simulink model "a1_walking_backward"  (R2022b)
settings: Solver=VariableStepAuto  StartTime=0.0  StopTime=5  RelTol=1e-3
values from neighbouring files (symbols this model uses):
  m = 12    [MPC_Controller.m]    (also in QP_Controller.m; TASK1_rotating_mpc.m; TASK1_walking_backward_mpc.m; TASK1_walking_forward_mpc.m)
  N = 10    [MPC_Controller.m]
undefined symbols (not defined in the file or in its folder): walking_forward_mpc, X, Y, Z
libraries: sm_lib x188, nesl_utility x120
(part 5 of 6)

== system a1_walking_backward/Rear Left Leg/RL_thigh ==
  Inertia : sm_lib/Body Elements/Inertia  InertiaType=Custom  Mass=1.013  MassUnits=kg  CenterOfMass=[0, 0, 0]  CenterOfMassUnits=m  MomentsOfInertia=[0.005529065, 0.005139339, 0.001367788]  MomentsOfInertiaUnits=kg*m^2  ProductsOfInertia=[2.2448e-05, 0.000343869, 4.825e-06]  ProductsOfInertiaUnits=kg*m^2  GraphicType=None  MarkerShape=Inertia  MarkerSize=20  GraphicVisPropType=SimpleVisualProperties  GraphicDiffuseColor=[0.5 0.5 0.5]  GraphicSpecularColor=[0.5 0.5 0.5 1.0]  GraphicAmbientColor=[0.15 0.15 0.15 1.0]  GraphicEmissiveColor=[0.0 0.0 0.0 1.0]  GraphicShininess=75  GraphicOpacity=1.0
  InertiaOriginTransform : sm_lib/Frames and Transforms/Rigid Transform  TranslationMethod=Cartesian  TranslationStandardOffset=0  TranslationLengthUnit=m  TranslationStandardAxis=+Z  TranslationCartesianOffset=[-0.003237, -0.022327, -0.027326]  TranslationROffset=0  TranslationROffsetUnits=m  TranslationZOffset=0  TranslationZOffsetUnits=m  TranslationThetaOffset=0  TranslationThetaOffsetUnits=deg  RotationMethod=RotationSequence  RotationAngleUnits=deg  RotationStandardAxis=+Z  RotationAngle=0.0  RotationArbitraryAxis=[0 0 1]  FollAlignAxisA=+X  BaseAlignAxisA=+Y  FollAlignAxisB=+Y  BaseAlignAxisB=+Z  RotationSequenceAxes=BaseAxes  RotationSequence=XYZ  RotationSequenceAngles=[0, 0, 0]  RotationSequenceAnglesUnits=rad  RotationMatrix=[1 0 0; 0 1 0; 0 0 1]  Quaternion=[1 0 0 0]
  RL_calf_joint_AxisTransform : sm_lib/Frames and Transforms/Rigid Transform  TranslationMethod=Cartesian  TranslationStandardOffset=0  TranslationLengthUnit=m  TranslationStandardAxis=+Z  TranslationCartesianOffset=[0, 0, 0]  TranslationROffset=0  TranslationROffsetUnits=m  TranslationZOffset=0  TranslationZOffsetUnits=m  TranslationThetaOffset=0  TranslationThetaOffsetUnits=deg  RotationMethod=ArbitraryAxis  RotationAngleUnits=rad  RotationStandardAxis=+Z  RotationAngle=1.570796326794897  RotationArbitraryAxis=[-1, 0, 0]  FollAlignAxisA=+X  BaseAlignAxisA=+Y  FollAlignAxisB=+Y  BaseAlignAxisB=+Z  RotationSequenceAxes=FollowerAxes  RotationSequence=XYX  RotationSequenceAngles=[0 0 0]  RotationSequenceAnglesUnits=deg  RotationMatrix=[1 0 0; 0 1 0; 0 0 1]  Quaternion=[1 0 0 0]
  RL_calf_joint_OriginTransform : sm_lib/Frames and Transforms/Rigid Transform  TranslationMethod=Cartesian  TranslationStandardOffset=0  TranslationLengthUnit=m  TranslationStandardAxis=+Z  TranslationCartesianOffset=[0, 0, -0.2]  TranslationROffset=0  TranslationROffsetUnits=m  TranslationZOffset=0  TranslationZOffsetUnits=m  TranslationThetaOffset=0  TranslationThetaOffsetUnits=deg  RotationMethod=RotationSequence  RotationAngleUnits=deg  RotationStandardAxis=+Z  RotationAngle=0.0  RotationArbitraryAxis=[0 0 1]  FollAlignAxisA=+X  BaseAlignAxisA=+Y  FollAlignAxisB=+Y  BaseAlignAxisB=+Z  RotationSequenceAxes=BaseAxes  RotationSequence=XYZ  RotationSequenceAngles=[0, 0, 0]  RotationSequenceAnglesUnits=rad  RotationMatrix=[1 0 0; 0 1 0; 0 0 1]  Quaternion=[1 0 0 0]
  RL_thigh_joint_AxisInvTransform : sm_lib/Frames and Transforms/Rigid Transform  TranslationMethod=Cartesian  TranslationStandardOffset=0  TranslationLengthUnit=m  TranslationStandardAxis=+Z  TranslationCartesianOffset=[0, 0, 0]  TranslationROffset=0  TranslationROffsetUnits=m  TranslationZOffset=0  TranslationZOffsetUnits=m  TranslationThetaOffset=0  TranslationThetaOffsetUnits=deg  RotationMethod=ArbitraryAxis  RotationAngleUnits=rad  RotationStandardAxis=+Z  RotationAngle=1.570796326794897  RotationArbitraryAxis=[-1, 0, 0]  FollAlignAxisA=+X  BaseAlignAxisA=+Y  FollAlignAxisB=+Y  BaseAlignAxisB=+Z  RotationSequenceAxes=FollowerAxes  RotationSequence=XYX  RotationSequenceAngles=[0 0 0]  RotationSequenceAnglesUnits=deg  RotationMatrix=[1 0 0; 0 1 0; 0 0 1]  Quaternion=[1 0 0 0]
  ReferenceFrame : sm_lib/Frames and Transforms/Reference Frame
  Visual : sm_lib/Body Elements/File Solid  ExtGeomFileName=AME556_project/a1_description/meshes/thigh.stl  UnitType=Custom  ExtGeomFileUnits=m  StepReaderType=HEX  ExportConvexHullGeometry=on  InertiaType=Custom  Mass=0  MassUnits=kg  CenterOfMass=[0, 0, 0]  CenterOfMassUnits=m  MomentsOfInertia=[0, 0, 0]  MomentsOfInertiaUnits=kg*m^2  ProductsOfInertia=[0, 0, 0]  ProductsOfInertiaUnits=kg*m^2  BasedOnType=DensityFromFile  Density=1000  DensityUnits=kg/m^3  DoExposeReferenceFrame=on  SerializedFrames=<Frames/>  GraphicType=FromGeometry  MarkerShape=Sphere  MarkerSize=10  GraphicVisPropType=SimpleVisualProperties  GraphicDiffuseColor=[1, 0.423529411765, 0.0392156862745]  GraphicSpecularColor=[0.5 0.5 0.5 1.0]  GraphicAmbientColor=[0.15 0.15 0.15 1.0]  GraphicEmissiveColor=[0.0 0.0 0.0 1.0]  GraphicShininess=75  GraphicOpacity=1
  VisualOriginTransform : sm_lib/Frames and Transforms/Rigid Transform  TranslationMethod=Cartesian  TranslationStandardOffset=0  TranslationLengthUnit=m  TranslationStandardAxis=+Z  TranslationCartesianOffset=[0, 0, 0]  TranslationROffset=0  TranslationROffsetUnits=m  TranslationZOffset=0  TranslationZOffsetUnits=m  TranslationThetaOffset=0  TranslationThetaOffsetUnits=deg  RotationMethod=RotationSequence  RotationAngleUnits=deg  RotationStandardAxis=+Z  RotationAngle=0.0  RotationArbitraryAxis=[0 0 1]  FollAlignAxisA=+X  BaseAlignAxisA=+Y  FollAlignAxisB=+Y  BaseAlignAxisB=+Z  RotationSequenceAxes=BaseAxes  RotationSequence=XYZ  RotationSequenceAngles=[0, 0, 0]  RotationSequenceAnglesUnits=rad  RotationMatrix=[1 0 0; 0 1 0; 0 0 1]  Quaternion=[1 0 0 0]
  F : PMIOPort  Side=Left
  F1 : PMIOPort  Port=2  Side=Right
  G : PMIOPort  Port=3  Side=Right
  connections:
  Inertia/RConn1 -- InertiaOriginTransform/RConn1
  RL_calf_joint_AxisTransform/RConn1 -- F1/RConn1
  RL_calf_joint_AxisTransform/LConn1 -- RL_calf_joint_OriginTransform/RConn1
  RL_thigh_joint_AxisInvTransform/RConn1 -- F/RConn1
  RL_calf_joint_OriginTransform/LConn1 -- InertiaOriginTransform/LConn1 -- ReferenceFrame/RConn1 -- VisualOriginTransform/LConn1 -- RL_thigh_joint_AxisInvTransform/LConn1
  Visual/RConn1 -- VisualOriginTransform/RConn1
  G/RConn1 -- Visual/LConn1

== system a1_walking_backward/Rear Left Leg/RL_thigh_shoulder ==
  ReferenceFrame : sm_lib/Frames and Transforms/Reference Frame
  F : PMIOPort  Side=Left
  connections:
  ReferenceFrame/RConn1 -- F/RConn1

== system a1_walking_backward/Rear Right Leg/Leg Logger11 ==
  PS-Simulink Converter : nesl_utility/PS-Simulink Converter  PhysicalDomain=network_engine_domain  SubClassName=ps_output  LeftPortType=input  RightPortType=output  PseudoPeriodic=off  Frequencies=[]  VectorFormat=inherit  Unit=inherit  AffineConversion=off
  PS-Simulink Converter1 : nesl_utility/PS-Simulink Converter  PhysicalDomain=network_engine_domain  SubClassName=ps_output  LeftPortType=input  RightPortType=output  PseudoPeriodic=off  Frequencies=[]  VectorFormat=inherit  Unit=inherit  AffineConversion=off
  PS-Simulink Converter2 : nesl_utility/PS-Simulink Converter  PhysicalDomain=network_engine_domain  SubClassName=ps_output  LeftPortType=input  RightPortType=output  PseudoPeriodic=off  Frequencies=[]  VectorFormat=inherit  Unit=inherit  AffineConversion=off
  Scope : Scope  NumInputPorts=3
  angle : PMIOPort  Side=Left
  velocity : PMIOPort  Port=2  Side=Left
  torque : PMIOPort  Port=3  Side=Left
  wires:
  PS-Simulink Converter/1 -> Scope/1  "RR_hip_joint angle (rad)"
  PS-Simulink Converter2/1 -> Scope/3  "RR_hip_joint torque (Nm)"
  PS-Simulink Converter1/1 -> Scope/2  "RR_hip_joint velocity (rad/s)"
  connections:
  PS-Simulink Converter2/LConn1 -- torque/RConn1
  PS-Simulink Converter/LConn1 -- angle/RConn1
  PS-Simulink Converter1/LConn1 -- velocity/RConn1

== system a1_walking_backward/Rear Right Leg/Leg Logger3 ==
  PS-Simulink Converter : nesl_utility/PS-Simulink Converter  PhysicalDomain=network_engine_domain  SubClassName=ps_output  LeftPortType=input  RightPortType=output  PseudoPeriodic=off  Frequencies=[]  VectorFormat=inherit  Unit=inherit  AffineConversion=off
  PS-Simulink Converter1 : nesl_utility/PS-Simulink Converter  PhysicalDomain=network_engine_domain  SubClassName=ps_output  LeftPortType=input  RightPortType=output  PseudoPeriodic=off  Frequencies=[]  VectorFormat=inherit  Unit=inherit  AffineConversion=off
  PS-Simulink Converter2 : nesl_utility/PS-Simulink Converter  PhysicalDomain=network_engine_domain  SubClassName=ps_output  LeftPortType=input  RightPortType=output  PseudoPeriodic=off  Frequencies=[]  VectorFormat=inherit  Unit=inherit  AffineConversion=off
  Scope : Scope  NumInputPorts=3
  angle : PMIOPort  Side=Left
  velocity : PMIOPort  Port=2  Side=Left
  torque : PMIOPort  Port=3  Side=Left
  wires:
  PS-Simulink Converter/1 -> Scope/1  "RR_calf_joint angle (rad)"
  PS-Simulink Converter2/1 -> Scope/3  "RR_calf_joint torque (Nm)"
  PS-Simulink Converter1/1 -> Scope/2  "RR_calf_joint velocity (rad/s)"
  connections:
  PS-Simulink Converter2/LConn1 -- torque/RConn1
  PS-Simulink Converter/LConn1 -- angle/RConn1
  PS-Simulink Converter1/LConn1 -- velocity/RConn1

== system a1_walking_backward/Rear Right Leg/Leg Logger4 ==
  PS-Simulink Converter : nesl_utility/PS-Simulink Converter  PhysicalDomain=network_engine_domain  SubClassName=ps_output  LeftPortType=input  RightPortType=output  PseudoPeriodic=off  Frequencies=[]  VectorFormat=inherit  Unit=inherit  AffineConversion=off
  PS-Simulink Converter1 : nesl_utility/PS-Simulink Converter  PhysicalDomain=network_engine_domain  SubClassName=ps_output  LeftPortType=input  RightPortType=output  PseudoPeriodic=off  Frequencies=[]  VectorFormat=inherit  Unit=inherit  AffineConversion=off
  PS-Simulink Converter2 : nesl_utility/PS-Simulink Converter  PhysicalDomain=network_engine_domain  SubClassName=ps_output  LeftPortType=input  RightPortType=output  PseudoPeriodic=off  Frequencies=[]  VectorFormat=inherit  Unit=inherit  AffineConversion=off
  Scope : Scope  NumInputPorts=3
  angle : PMIOPort  Side=Left
  velocity : PMIOPort  Port=2  Side=Left
  torque : PMIOPort  Port=3  Side=Left
  wires:
  PS-Simulink Converter/1 -> Scope/1  "RR_thigh_joint angle (rad)"
  PS-Simulink Converter2/1 -> Scope/3  "RR_thigh_joint torque (Nm)"
  PS-Simulink Converter1/1 -> Scope/2  "RR_thigh_joint velocity (rad/s)"
  connections:
  PS-Simulink Converter2/LConn1 -- torque/RConn1
  PS-Simulink Converter/LConn1 -- angle/RConn1
  PS-Simulink Converter1/LConn1 -- velocity/RConn1

== system a1_walking_backward/Rear Right Leg/RR_calf ==
  Inertia : sm_lib/Body Elements/Inertia  InertiaType=Custom  Mass=0.166  MassUnits=kg  CenterOfMass=[0, 0, 0]  CenterOfMassUnits=m  MomentsOfInertia=[0.002997972, 0.003014022, 3.2426e-05]  MomentsOfInertiaUnits=kg*m^2  ProductsOfInertia=[0, -0.000141163, 0]  ProductsOfInertiaUnits=kg*m^2  GraphicType=None  MarkerShape=Inertia  MarkerSize=20  GraphicVisPropType=SimpleVisualProperties  GraphicDiffuseColor=[0.5 0.5 0.5]  GraphicSpecularColor=[0.5 0.5 0.5 1.0]  GraphicAmbientColor=[0.15 0.15 0.15 1.0]  GraphicEmissiveColor=[0.0 0.0 0.0 1.0]  GraphicShininess=75  GraphicOpacity=1.0
  InertiaOriginTransform : sm_lib/Frames and Transforms/Rigid Transform  TranslationMethod=Cartesian  TranslationStandardOffset=0  TranslationLengthUnit=m  TranslationStandardAxis=+Z  TranslationCartesianOffset=[0.006435, 0, -0.107388]  TranslationROffset=0  TranslationROffsetUnits=m  TranslationZOffset=0  TranslationZOffsetUnits=m  TranslationThetaOffset=0  TranslationThetaOffsetUnits=deg  RotationMethod=RotationSequence  RotationAngleUnits=deg  RotationStandardAxis=+Z  RotationAngle=0.0  RotationArbitraryAxis=[0 0 1]  FollAlignAxisA=+X  BaseAlignAxisA=+Y  FollAlignAxisB=+Y  BaseAlignAxisB=+Z  RotationSequenceAxes=BaseAxes  RotationSequence=XYZ  RotationSequenceAngles=[0, 0, 0]  RotationSequenceAnglesUnits=rad  RotationMatrix=[1 0 0; 0 1 0; 0 0 1]  Quaternion=[1 0 0 0]
  RR_calf_joint_AxisInvTransform : sm_lib/Frames and Transforms/Rigid Transform  TranslationMethod=Cartesian  TranslationStandardOffset=0  TranslationLengthUnit=m  TranslationStandardAxis=+Z  TranslationCartesianOffset=[0, 0, 0]  TranslationROffset=0  TranslationROffsetUnits=m  TranslationZOffset=0  TranslationZOffsetUnits=m  TranslationThetaOffset=0  TranslationThetaOffsetUnits=deg  RotationMethod=ArbitraryAxis  RotationAngleUnits=rad  RotationStandardAxis=+Z  RotationAngle=1.570796326794897  RotationArbitraryAxis=[-1, 0, 0]  FollAlignAxisA=+X  BaseAlignAxisA=+Y  FollAlignAxisB=+Y  BaseAlignAxisB=+Z  RotationSequenceAxes=FollowerAxes  RotationSequence=XYX  RotationSequenceAngles=[0 0 0]  RotationSequenceAnglesUnits=deg  RotationMatrix=[1 0 0; 0 1 0; 0 0 1]  Quaternion=[1 0 0 0]
  RR_foot_fixed_OriginTransform : sm_lib/Frames and Transforms/Rigid Transform  TranslationMethod=Cartesian  TranslationStandardOffset=0  TranslationLengthUnit=m  TranslationStandardAxis=+Z  TranslationCartesianOffset=[0, 0, -0.2]  TranslationROffset=0  TranslationROffsetUnits=m  TranslationZOffset=0  TranslationZOffsetUnits=m  TranslationThetaOffset=0  TranslationThetaOffsetUnits=deg  RotationMethod=RotationSequence  RotationAngleUnits=deg  RotationStandardAxis=+Z  RotationAngle=0.0  RotationArbitraryAxis=[0 0 1]  FollAlignAxisA=+X  BaseAlignAxisA=+Y  FollAlignAxisB=+Y  BaseAlignAxisB=+Z  RotationSequenceAxes=BaseAxes  RotationSequence=XYZ  RotationSequenceAngles=[0, 0, 0]  RotationSequenceAnglesUnits=rad  RotationMatrix=[1 0 0; 0 1 0; 0 0 1]  Quaternion=[1 0 0 0]
  ReferenceFrame : sm_lib/Frames and Transforms/Reference Frame
  Visual : sm_lib/Body Elements/File Solid  ExtGeomFileName=AME556_project/a1_description/meshes/calf.stl  UnitType=Custom  ExtGeomFileUnits=m  StepReaderType=HEX  ExportConvexHullGeometry=off  InertiaType=Custom  Mass=0  MassUnits=kg  CenterOfMass=[0, 0, 0]  CenterOfMassUnits=m  MomentsOfInertia=[0, 0, 0]  MomentsOfInertiaUnits=kg*m^2  ProductsOfInertia=[0, 0, 0]  ProductsOfInertiaUnits=kg*m^2  BasedOnType=DensityFromFile  Density=1000  DensityUnits=kg/m^3  DoExposeReferenceFrame=on  SerializedFrames=<Frames/>  GraphicType=FromGeometry  MarkerShape=Sphere  MarkerSize=10  GraphicVisPropType=SimpleVisualProperties  GraphicDiffuseColor=[1, 0.423529411765, 0.0392156862745]  GraphicSpecularColor=[0.5 0.5 0.5 1.0]  GraphicAmbientColor=[0.15 0.15 0.15 1.0]  GraphicEmissiveColor=[0.0 0.0 0.0 1.0]  GraphicShininess=75  GraphicOpacity=1
  VisualOriginTransform : sm_lib/Frames and Transforms/Rigid Transform  TranslationMethod=Cartesian  TranslationStandardOffset=0  TranslationLengthUnit=m  TranslationStandardAxis=+Z  TranslationCartesianOffset=[0, 0, 0]  TranslationROffset=0  TranslationROffsetUnits=m  TranslationZOffset=0  TranslationZOffsetUnits=m  TranslationThetaOffset=0  TranslationThetaOffsetUnits=deg  RotationMethod=RotationSequence  RotationAngleUnits=deg  RotationStandardAxis=+Z  RotationAngle=0.0  RotationArbitraryAxis=[0 0 1]  FollAlignAxisA=+X  BaseAlignAxisA=+Y  FollAlignAxisB=+Y  BaseAlignAxisB=+Z  RotationSequenceAxes=BaseAxes  RotationSequence=XYZ  RotationSequenceAngles=[0, 0, 0]  RotationSequenceAnglesUnits=rad  RotationMatrix=[1 0 0; 0 1 0; 0 0 1]  Quaternion=[1 0 0 0]
  F : PMIOPort  Side=Left
  F1 : PMIOPort  Port=2  Side=Right
  connections:
  Inertia/RConn1 -- InertiaOriginTransform/RConn1
  RR_calf_joint_AxisInvTransform/RConn1 -- F/RConn1
  RR_foot_fixed_OriginTransform/RConn1 -- F1/RConn1
  RR_calf_joint_AxisInvTransform/LConn1 -- InertiaOriginTransform/LConn1 -- ReferenceFrame/RConn1 -- VisualOriginTransform/LConn1 -- RR_foot_fixed_OriginTransform/LConn1
  Visual/RConn1 -- VisualOriginTransform/RConn1

== system a1_walking_backward/Rear Right Leg/RR_foot ==
  Inertia : sm_lib/Body Elements/Inertia  InertiaType=Custom  Mass=0.06  MassUnits=kg  CenterOfMass=[0, 0, 0]  CenterOfMassUnits=m  MomentsOfInertia=[9.6e-06, 9.6e-06, 9.6e-06]  MomentsOfInertiaUnits=kg*m^2  ProductsOfInertia=[0, 0, 0]  ProductsOfInertiaUnits=kg*m^2  GraphicType=None  MarkerShape=Inertia  MarkerSize=20  GraphicVisPropType=SimpleVisualProperties  GraphicDiffuseColor=[0.5 0.5 0.5]  GraphicSpecularColor=[0.5 0.5 0.5 1.0]  GraphicAmbientColor=[0.15 0.15 0.15 1.0]  GraphicEmissiveColor=[0.0 0.0 0.0 1.0]  GraphicShininess=75  GraphicOpacity=1.0
  InertiaOriginTransform : sm_lib/Frames and Transforms/Rigid Transform  TranslationMethod=Cartesian  TranslationStandardOffset=0  TranslationLengthUnit=m  TranslationStandardAxis=+Z  TranslationCartesianOffset=[0, 0, 0]  TranslationROffset=0  TranslationROffsetUnits=m  TranslationZOffset=0  TranslationZOffsetUnits=m  TranslationThetaOffset=0  TranslationThetaOffsetUnits=deg  RotationMethod=RotationSequence  RotationAngleUnits=deg  RotationStandardAxis=+Z  RotationAngle=0.0  RotationArbitraryAxis=[0 0 1]  FollAlignAxisA=+X  BaseAlignAxisA=+Y  FollAlignAxisB=+Y  BaseAlignAxisB=+Z  RotationSequenceAxes=BaseAxes  RotationSequence=XYZ  RotationSequenceAngles=[0, 0, 0]  RotationSequenceAnglesUnits=rad  RotationMatrix=[1 0 0; 0 1 0; 0 0 1]  Quaternion=[1 0 0 0]
  ReferenceFrame : sm_lib/Frames and Transforms/Reference Frame
  Visual : sm_lib/Body Elements/Spherical Solid  GraphicAmbientColor=[0.15 0.15 0.15 1.0]  BasedOnType=Density  CenterOfMass=[0, 0, 0]  CenterOfMassUnits=m  GraphicDiffuseColor=[1, 0.423529411765, 0.0392156862745]  Density=1000  DensityUnits=kg/m^3  DoExposeReferenceFrame=on  GraphicEmissiveColor=[0.0 0.0 0.0 1.0]  ExportEntireGeometry=on  SerializedExposedGeometries=<ExposedGeometries><ExposedGeometry><RawGeometryId>entire</RawGeometryId><ExposedGeometryId>G</ExposedGeometryId></ExposedGeometry></ExposedGeometries>  SerializedFrames=<Frames/>  MarkerShape=Sphere  MarkerSize=10  GraphicType=FromGeometry  InertiaType=Custom  Mass=0  MassUnits=kg  MomentsOfInertia=[0, 0, 0]  MomentsOfInertiaUnits=kg*m^2  GraphicOpacity=1  ProductsOfInertia=[0, 0, 0]  ProductsOfInertiaUnits=kg*m^2  GraphicShininess=75  GraphicSpecularColor=[0.5 0.5 0.5 1.0]  SphereRadius=0.01  SphereRadiusUnits=m  GraphicVisPropType=SimpleVisualProperties
  VisualOriginTransform : sm_lib/Frames and Transforms/Rigid Transform  TranslationMethod=Cartesian  TranslationStandardOffset=0  TranslationLengthUnit=m  TranslationStandardAxis=+Z  TranslationCartesianOffset=[0, 0, 0]  TranslationROffset=0  TranslationROffsetUnits=m  TranslationZOffset=0  TranslationZOffsetUnits=m  TranslationThetaOffset=0  TranslationThetaOffsetUnits=deg  RotationMethod=RotationSequence  RotationAngleUnits=deg  RotationStandardAxis=+Z  RotationAngle=0.0  RotationArbitraryAxis=[0 0 1]  FollAlignAxisA=+X  BaseAlignAxisA=+Y  FollAlignAxisB=+Y  BaseAlignAxisB=+Z  RotationSequenceAxes=BaseAxes  RotationSequence=XYZ  RotationSequenceAngles=[0, 0, 0]  RotationSequenceAnglesUnits=rad  RotationMatrix=[1 0 0; 0 1 0; 0 0 1]  Quaternion=[1 0 0 0]
  F : PMIOPort  Side=Left
  G : PMIOPort  Port=2  Side=Left
  connections:
  Inertia/RConn1 -- InertiaOriginTransform/RConn1
  ReferenceFrame/RConn1 -- InertiaOriginTransform/LConn1 -- VisualOriginTransform/LConn1 -- F/RConn1
  Visual/RConn1 -- VisualOriginTransform/RConn1
  G/RConn1 -- Visual/LConn1

== system a1_walking_backward/Rear Right Leg/RR_hip ==
  Inertia : sm_lib/Body Elements/Inertia  InertiaType=Custom  Mass=0.696  MassUnits=kg  CenterOfMass=[0, 0, 0]  CenterOfMassUnits=m  MomentsOfInertia=[0.000469246, 0.00080749, 0.000552929]  MomentsOfInertiaUnits=kg*m^2  ProductsOfInertia=[4.66e-07, 3.42e-07, -9.408999999999999e-06]  ProductsOfInertiaUnits=kg*m^2  GraphicType=None  MarkerShape=Inertia  MarkerSize=20  GraphicVisPropType=SimpleVisualProperties  GraphicDiffuseColor=[0.5 0.5 0.5]  GraphicSpecularColor=[0.5 0.5 0.5 1.0]  GraphicAmbientColor=[0.15 0.15 0.15 1.0]  GraphicEmissiveColor=[0.0 0.0 0.0 1.0]  GraphicShininess=75  GraphicOpacity=1.0
  InertiaOriginTransform : sm_lib/Frames and Transforms/Rigid Transform  TranslationMethod=Cartesian  TranslationStandardOffset=0  TranslationLengthUnit=m  TranslationStandardAxis=+Z  TranslationCartesianOffset=[0.003311, -0.000635, 3.1e-05]  TranslationROffset=0  TranslationROffsetUnits=m  TranslationZOffset=0  TranslationZOffsetUnits=m  TranslationThetaOffset=0  TranslationThetaOffsetUnits=deg  RotationMethod=RotationSequence  RotationAngleUnits=deg  RotationStandardAxis=+Z  RotationAngle=0.0  RotationArbitraryAxis=[0 0 1]  FollAlignAxisA=+X  BaseAlignAxisA=+Y  FollAlignAxisB=+Y  BaseAlignAxisB=+Z  RotationSequenceAxes=BaseAxes  RotationSequence=XYZ  RotationSequenceAngles=[0, 0, 0]  RotationSequenceAnglesUnits=rad  RotationMatrix=[1 0 0; 0 1 0; 0 0 1]  Quaternion=[1 0 0 0]
  RR_hip_fixed_OriginTransform : sm_lib/Frames and Transforms/Rigid Transform  TranslationMethod=Cartesian  TranslationStandardOffset=0  TranslationLengthUnit=m  TranslationStandardAxis=+Z  TranslationCartesianOffset=[0, -0.081, 0]  TranslationROffset=0  TranslationROffsetUnits=m  TranslationZOffset=0  TranslationZOffsetUnits=m  TranslationThetaOffset=0  TranslationThetaOffsetUnits=deg  RotationMethod=RotationSequence  RotationAngleUnits=deg  RotationStandardAxis=+Z  RotationAngle=0.0  RotationArbitraryAxis=[0 0 1]  FollAlignAxisA=+X  BaseAlignAxisA=+Y  FollAlignAxisB=+Y  BaseAlignAxisB=+Z  RotationSequenceAxes=BaseAxes  RotationSequence=XYZ  RotationSequenceAngles=[0, 0, 0]  RotationSequenceAnglesUnits=rad  RotationMatrix=[1 0 0; 0 1 0; 0 0 1]  Quaternion=[1 0 0 0]
  RR_hip_joint_AxisInvTransform : sm_lib/Frames and Transforms/Rigid Transform  TranslationMethod=Cartesian  TranslationStandardOffset=0  TranslationLengthUnit=m  TranslationStandardAxis=+Z  TranslationCartesianOffset=[0, 0, 0]  TranslationROffset=0  TranslationROffsetUnits=m  TranslationZOffset=0  TranslationZOffsetUnits=m  TranslationThetaOffset=0  TranslationThetaOffsetUnits=deg  RotationMethod=ArbitraryAxis  RotationAngleUnits=rad  RotationStandardAxis=+Z  RotationAngle=1.570796326794897  RotationArbitraryAxis=[-0, 1, 0]  FollAlignAxisA=+X  BaseAlignAxisA=+Y  FollAlignAxisB=+Y  BaseAlignAxisB=+Z  RotationSequenceAxes=FollowerAxes  RotationSequence=XYX  RotationSequenceAngles=[0 0 0]  RotationSequenceAnglesUnits=deg  RotationMatrix=[1 0 0; 0 1 0; 0 0 1]  Quaternion=[1 0 0 0]
  RR_thigh_joint_AxisTransform : sm_lib/Frames and Transforms/Rigid Transform  TranslationMethod=Cartesian  TranslationStandardOffset=0  TranslationLengthUnit=m  TranslationStandardAxis=+Z  TranslationCartesianOffset=[0, 0, 0]  TranslationROffset=0  TranslationROffsetUnits=m  TranslationZOffset=0  TranslationZOffsetUnits=m  TranslationThetaOffset=0  TranslationThetaOffsetUnits=deg  RotationMethod=ArbitraryAxis  RotationAngleUnits=rad  RotationStandardAxis=+Z  RotationAngle=1.570796326794897  RotationArbitraryAxis=[-1, 0, 0]  FollAlignAxisA=+X  BaseAlignAxisA=+Y  FollAlignAxisB=+Y  BaseAlignAxisB=+Z  RotationSequenceAxes=FollowerAxes  RotationSequence=XYX  RotationSequenceAngles=[0 0 0]  RotationSequenceAnglesUnits=deg  RotationMatrix=[1 0 0; 0 1 0; 0 0 1]  Quaternion=[1 0 0 0]
  RR_thigh_joint_OriginTransform : sm_lib/Frames and Transforms/Rigid Transform  TranslationMethod=Cartesian  TranslationStandardOffset=0  TranslationLengthUnit=m  TranslationStandardAxis=+Z  TranslationCartesianOffset=[0, -0.0838, 0]  TranslationROffset=0  TranslationROffsetUnits=m  TranslationZOffset=0  TranslationZOffsetUnits=m  TranslationThetaOffset=0  TranslationThetaOffsetUnits=deg  RotationMethod=RotationSequence  RotationAngleUnits=deg  RotationStandardAxis=+Z  RotationAngle=0.0  RotationArbitraryAxis=[0 0 1]  FollAlignAxisA=+X  BaseAlignAxisA=+Y  FollAlignAxisB=+Y  BaseAlignAxisB=+Z  RotationSequenceAxes=BaseAxes  RotationSequence=XYZ  RotationSequenceAngles=[0, 0, 0]  RotationSequenceAnglesUnits=rad  RotationMatrix=[1 0 0; 0 1 0; 0 0 1]  Quaternion=[1 0 0 0]
  ReferenceFrame : sm_lib/Frames and Transforms/Reference Frame
  Visual : sm_lib/Body Elements/File Solid  ExtGeomFileName=AME556_project/a1_description/meshes/hip.stl  UnitType=Custom  ExtGeomFileUnits=m  StepReaderType=HEX  ExportConvexHullGeometry=off  InertiaType=Custom  Mass=0  MassUnits=kg  CenterOfMass=[0, 0, 0]  CenterOfMassUnits=m  MomentsOfInertia=[0, 0, 0]  MomentsOfInertiaUnits=kg*m^2  ProductsOfInertia=[0, 0, 0]  ProductsOfInertiaUnits=kg*m^2  BasedOnType=DensityFromFile  Density=1000  DensityUnits=kg/m^3  DoExposeReferenceFrame=on  SerializedFrames=<Frames/>  GraphicType=FromGeometry  MarkerShape=Sphere  MarkerSize=10  GraphicVisPropType=SimpleVisualProperties  GraphicDiffuseColor=[1, 0.423529411765, 0.0392156862745]  GraphicSpecularColor=[0.5 0.5 0.5 1.0]  GraphicAmbientColor=[0.15 0.15 0.15 1.0]  GraphicEmissiveColor=[0.0 0.0 0.0 1.0]  GraphicShininess=75  GraphicOpacity=1
  VisualOriginTransform : sm_lib/Frames and Transforms/Rigid Transform  TranslationMethod=Cartesian  TranslationStandardOffset=0  TranslationLengthUnit=m  TranslationStandardAxis=+Z  TranslationCartesianOffset=[0, 0, 0]  TranslationROffset=0  TranslationROffsetUnits=m  TranslationZOffset=0  TranslationZOffsetUnits=m  TranslationThetaOffset=0  TranslationThetaOffsetUnits=deg  RotationMethod=RotationSequence  RotationAngleUnits=deg  RotationStandardAxis=+Z  RotationAngle=0.0  RotationArbitraryAxis=[0 0 1]  FollAlignAxisA=+X  BaseAlignAxisA=+Y  FollAlignAxisB=+Y  BaseAlignAxisB=+Z  RotationSequenceAxes=BaseAxes  RotationSequence=XYZ  RotationSequenceAngles=[3.14159265359, 3.14159265359, 0]  RotationSequenceAnglesUnits=rad  RotationMatrix=[1 0 0; 0 1 0; 0 0 1]  Quaternion=[1 0 0 0]
  F : PMIOPort  Side=Left
  F2 : PMIOPort  Port=2  Side=Right
  F1 : PMIOPort  Port=3  Side=Right
  connections:
  Inertia/RConn1 -- InertiaOriginTransform/RConn1
  RR_hip_fixed_OriginTransform/RConn1 -- F1/RConn1
  RR_hip_joint_AxisInvTransform/RConn1 -- F/RConn1
  RR_thigh_joint_AxisTransform/RConn1 -- F2/RConn1
  RR_thigh_joint_AxisTransform/LConn1 -- RR_thigh_joint_OriginTransform/RConn1
  RR_hip_fixed_OriginTransform/LConn1 -- RR_hip_joint_AxisInvTransform/LConn1 -- RR_thigh_joint_OriginTransform/LConn1 -- InertiaOriginTransform/LConn1 -- ReferenceFrame/RConn1 -- VisualOriginTransform/LConn1
  Visual/RConn1 -- VisualOriginTransform/RConn1

== system a1_walking_backward/Rear Right Leg/RR_thigh ==
  Inertia : sm_lib/Body Elements/Inertia  InertiaType=Custom  Mass=1.013  MassUnits=kg  CenterOfMass=[0, 0, 0]  CenterOfMassUnits=m  MomentsOfInertia=[0.005529065, 0.005139339, 0.001367788]  MomentsOfInertiaUnits=kg*m^2  ProductsOfInertia=[-2.2448e-05, 0.000343869, -4.825e-06]  ProductsOfInertiaUnits=kg*m^2  GraphicType=None  MarkerShape=Inertia  MarkerSize=20  GraphicVisPropType=SimpleVisualProperties  GraphicDiffuseColor=[0.5 0.5 0.5]  GraphicSpecularColor=[0.5 0.5 0.5 1.0]  GraphicAmbientColor=[0.15 0.15 0.15 1.0]  GraphicEmissiveColor=[0.0 0.0 0.0 1.0]  GraphicShininess=75  GraphicOpacity=1.0
  InertiaOriginTransform : sm_lib/Frames and Transforms/Rigid Transform  TranslationMethod=Cartesian  TranslationStandardOffset=0  TranslationLengthUnit=m  TranslationStandardAxis=+Z  TranslationCartesianOffset=[-0.003237, 0.022327, -0.027326]  TranslationROffset=0  TranslationROffsetUnits=m  TranslationZOffset=0  TranslationZOffsetUnits=m  TranslationThetaOffset=0  TranslationThetaOffsetUnits=deg  RotationMethod=RotationSequence  RotationAngleUnits=deg  RotationStandardAxis=+Z  RotationAngle=0.0  RotationArbitraryAxis=[0 0 1]  FollAlignAxisA=+X  BaseAlignAxisA=+Y  FollAlignAxisB=+Y  BaseAlignAxisB=+Z  RotationSequenceAxes=BaseAxes  RotationSequence=XYZ  RotationSequenceAngles=[0, 0, 0]  RotationSequenceAnglesUnits=rad  RotationMatrix=[1 0 0; 0 1 0; 0 0 1]  Quaternion=[1 0 0 0]
  RR_calf_joint_AxisTransform : sm_lib/Frames and Transforms/Rigid Transform  TranslationMethod=Cartesian  TranslationStandardOffset=0  TranslationLengthUnit=m  TranslationStandardAxis=+Z  TranslationCartesianOffset=[0, 0, 0]  TranslationROffset=0  TranslationROffsetUnits=m  TranslationZOffset=0  TranslationZOffsetUnits=m  TranslationThetaOffset=0  TranslationThetaOffsetUnits=deg  RotationMethod=ArbitraryAxis  RotationAngleUnits=rad  RotationStandardAxis=+Z  RotationAngle=1.570796326794897  RotationArbitraryAxis=[-1, 0, 0]  FollAlignAxisA=+X  BaseAlignAxisA=+Y  FollAlignAxisB=+Y  BaseAlignAxisB=+Z  RotationSequenceAxes=FollowerAxes  RotationSequence=XYX  RotationSequenceAngles=[0 0 0]  RotationSequenceAnglesUnits=deg  RotationMatrix=[1 0 0; 0 1 0; 0 0 1]  Quaternion=[1 0 0 0]
  RR_calf_joint_OriginTransform : sm_lib/Frames and Transforms/Rigid Transform  TranslationMethod=Cartesian  TranslationStandardOffset=0  TranslationLengthUnit=m  TranslationStandardAxis=+Z  TranslationCartesianOffset=[0, 0, -0.2]  TranslationROffset=0  TranslationROffsetUnits=m  TranslationZOffset=0  TranslationZOffsetUnits=m  TranslationThetaOffset=0  TranslationThetaOffsetUnits=deg  RotationMethod=RotationSequence  RotationAngleUnits=deg  RotationStandardAxis=+Z  RotationAngle=0.0  RotationArbitraryAxis=[0 0 1]  FollAlignAxisA=+X  BaseAlignAxisA=+Y  FollAlignAxisB=+Y  BaseAlignAxisB=+Z  RotationSequenceAxes=BaseAxes  RotationSequence=XYZ  RotationSequenceAngles=[0, 0, 0]  RotationSequenceAnglesUnits=rad  RotationMatrix=[1 0 0; 0 1 0; 0 0 1]  Quaternion=[1 0 0 0]
  RR_thigh_joint_AxisInvTransform : sm_lib/Frames and Transforms/Rigid Transform  TranslationMethod=Cartesian  TranslationStandardOffset=0  TranslationLengthUnit=m  TranslationStandardAxis=+Z  TranslationCartesianOffset=[0, 0, 0]  TranslationROffset=0  TranslationROffsetUnits=m  TranslationZOffset=0  TranslationZOffsetUnits=m  TranslationThetaOffset=0  TranslationThetaOffsetUnits=deg  RotationMethod=ArbitraryAxis  RotationAngleUnits=rad  RotationStandardAxis=+Z  RotationAngle=1.570796326794897  RotationArbitraryAxis=[-1, 0, 0]  FollAlignAxisA=+X  BaseAlignAxisA=+Y  FollAlignAxisB=+Y  BaseAlignAxisB=+Z  RotationSequenceAxes=FollowerAxes  RotationSequence=XYX  RotationSequenceAngles=[0 0 0]  RotationSequenceAnglesUnits=deg  RotationMatrix=[1 0 0; 0 1 0; 0 0 1]  Quaternion=[1 0 0 0]
  ReferenceFrame : sm_lib/Frames and Transforms/Reference Frame
  Visual : sm_lib/Body Elements/File Solid  ExtGeomFileName=AME556_project/a1_description/meshes/thigh_mirror.stl  UnitType=Custom  ExtGeomFileUnits=m  StepReaderType=HEX  ExportConvexHullGeometry=on  InertiaType=Custom  Mass=0  MassUnits=kg  CenterOfMass=[0, 0, 0]  CenterOfMassUnits=m  MomentsOfInertia=[0, 0, 0]  MomentsOfInertiaUnits=kg*m^2  ProductsOfInertia=[0, 0, 0]  ProductsOfInertiaUnits=kg*m^2  BasedOnType=DensityFromFile  Density=1000  DensityUnits=kg/m^3  DoExposeReferenceFrame=on  SerializedFrames=<Frames/>  GraphicType=FromGeometry  MarkerShape=Sphere  MarkerSize=10  GraphicVisPropType=SimpleVisualProperties  GraphicDiffuseColor=[1, 0.423529411765, 0.0392156862745]  GraphicSpecularColor=[0.5 0.5 0.5 1.0]  GraphicAmbientColor=[0.15 0.15 0.15 1.0]  GraphicEmissiveColor=[0.0 0.0 0.0 1.0]  GraphicShininess=75  GraphicOpacity=1
  VisualOriginTransform : sm_lib/Frames and Transforms/Rigid Transform  TranslationMethod=Cartesian  TranslationStandardOffset=0  TranslationLengthUnit=m  TranslationStandardAxis=+Z  TranslationCartesianOffset=[0, 0, 0]  TranslationROffset=0  TranslationROffsetUnits=m  TranslationZOffset=0  TranslationZOffsetUnits=m  TranslationThetaOffset=0  TranslationThetaOffsetUnits=deg  RotationMethod=RotationSequence  RotationAngleUnits=deg  RotationStandardAxis=+Z  RotationAngle=0.0  RotationArbitraryAxis=[0 0 1]  FollAlignAxisA=+X  BaseAlignAxisA=+Y  FollAlignAxisB=+Y  BaseAlignAxisB=+Z  RotationSequenceAxes=BaseAxes  RotationSequence=XYZ  RotationSequenceAngles=[0, 0, 0]  RotationSequenceAnglesUnits=rad  RotationMatrix=[1 0 0; 0 1 0; 0 0 1]  Quaternion=[1 0 0 0]
  F : PMIOPort  Side=Left
  G : PMIOPort  Port=2  Side=Right
  F1 : PMIOPort  Port=3  Side=Right
  connections:
  Inertia/RConn1 -- InertiaOriginTransform/RConn1
  RR_calf_joint_AxisTransform/RConn1 -- F1/RConn1
  RR_calf_joint_AxisTransform/LConn1 -- RR_calf_joint_OriginTransform/RConn1
  RR_thigh_joint_AxisInvTransform/RConn1 -- F/RConn1
  RR_calf_joint_OriginTransform/LConn1 -- InertiaOriginTransform/LConn1 -- ReferenceFrame/RConn1 -- VisualOriginTransform/LConn1 -- RR_thigh_joint_AxisInvTransform/LConn1
  Visual/RConn1 -- VisualOriginTransform/RConn1
  G/RConn1 -- Visual/LConn1

== system a1_walking_backward/Rear Right Leg/RR_thigh_shoulder ==
  ReferenceFrame : sm_lib/Frames and Transforms/Reference Frame
  F : PMIOPort  Side=Left
  connections:
  ReferenceFrame/RConn1 -- F/RConn1

== system a1_walking_backward/Stand Controller/Subsystem1 ==
  angle : Inport
  velocity : Inport  Port=2
  Add : Sum
  Constant1 : Constant  Value=-2
  Constant2 : Constant  Value=-20
  Constant3 : Constant  Value=0.5
  Product : Product
  Product1 : Product
  Saturation : Saturate  UpperLimit=33.5  LowerLimit=-33.5
  Subtract : Sum  Inputs=+-
  Torque : Outport
  wires:
  angle/1 -> Subtract/1
  Constant2/1 -> Product/2
  Subtract/1 -> Product/1
  Constant1/1 -> Product1/2
  velocity/1 -> Product1/1
  Product1/1 -> Add/2
  Product/1 -> Add/1
  Constant3/1 -> Subtract/2
  Add/1 -> Saturation/1
  Saturation/1 -> Torque/1

== system a1_walking_backward/Stand Controller/Subsystem10 ==
  angle : Inport
  velocity : Inport  Port=2
  Add : Sum
  Constant1 : Constant  Value=-6
  Constant2 : Constant  Value=-60
  Constant3 : Constant  Value=0.8
  Product : Product
  Product1 : Product
  Saturation : Saturate  UpperLimit=33.5  LowerLimit=-33.5
  Subtract : Sum  Inputs=+-
  Torque : Outport
  wires:
  angle/1 -> Subtract/1
  Constant2/1 -> Product/2
  Subtract/1 -> Product/1
  Constant1/1 -> Product1/2
  velocity/1 -> Product1/1
  Product1/1 -> Add/2
  Product/1 -> Add/1
  Constant3/1 -> Subtract/2
  Add/1 -> Saturation/1
  Saturation/1 -> Torque/1

== system a1_walking_backward/Stand Controller/Subsystem11 ==
  angle : Inport
  velocity : Inport  Port=2
  Add : Sum
  Constant1 : Constant  Value=-4
  Constant2 : Constant  Value=-40
  Constant3 : Constant  Value=-1
  Product : Product
  Product1 : Product
  Saturation : Saturate  UpperLimit=33.5  LowerLimit=-33.5
  Subtract : Sum  Inputs=+-
  Torque : Outport
  wires:
  angle/1 -> Subtract/1
  Constant2/1 -> Product/2
  Subtract/1 -> Product/1
  Constant1/1 -> Product1/2
  velocity/1 -> Product1/1
  Product1/1 -> Add/2
  Product/1 -> Add/1
  Constant3/1 -> Subtract/2
  Add/1 -> Saturation/1
  Saturation/1 -> Torque/1

== system a1_walking_backward/Stand Controller/Subsystem12 ==
  angle : Inport
  velocity : Inport  Port=2
  Add : Sum
  Constant1 : Constant  Value=-2
  Constant2 : Constant  Value=-20
  Constant3 : Constant  Value=0
  Product : Product
  Product1 : Product
  Saturation : Saturate  UpperLimit=33.5  LowerLimit=-33.5
  Subtract : Sum  Inputs=+-
  Torque : Outport
  wires:
  angle/1 -> Subtract/1
  Constant2/1 -> Product/2
  Subtract/1 -> Product/1
  Constant1/1 -> Product1/2
  velocity/1 -> Product1/1
  Product1/1 -> Add/2
  Product/1 -> Add/1
  Constant3/1 -> Subtract/2
  Add/1 -> Saturation/1
  Saturation/1 -> Torque/1

== system a1_walking_backward/Stand Controller/Subsystem2 ==
  angle : Inport
  velocity : Inport  Port=2
  Add : Sum
  Constant1 : Constant  Value=-6
  Constant2 : Constant  Value=-60
  Constant3 : Constant  Value=0.8
  Product : Product
  Product1 : Product
  Saturation : Saturate  UpperLimit=33.5  LowerLimit=-33.5
  Subtract : Sum  Inputs=+-
  Torque : Outport
  wires:
  angle/1 -> Subtract/1
  Constant2/1 -> Product/2
  Subtract/1 -> Product/1
  Constant1/1 -> Product1/2
  velocity/1 -> Product1/1
  Product1/1 -> Add/2
  Product/1 -> Add/1
  Constant3/1 -> Subtract/2
  Add/1 -> Saturation/1
  Saturation/1 -> Torque/1

== system a1_walking_backward/Stand Controller/Subsystem3 ==
  angle : Inport
  velocity : Inport  Port=2
  Add : Sum
  Constant1 : Constant  Value=-2
  Constant2 : Constant  Value=-20
  Constant3 : Constant  Value=-1
  Product : Product
  Product1 : Product
  Saturation : Saturate  UpperLimit=33.5  LowerLimit=-33.5
  Subtract : Sum  Inputs=+-
  Torque : Outport
  wires:
  angle/1 -> Subtract/1
  Constant2/1 -> Product/2
  Subtract/1 -> Product/1
  Constant1/1 -> Product1/2
  velocity/1 -> Product1/1
  Product1/1 -> Add/2
  Product/1 -> Add/1
  Constant3/1 -> Subtract/2
  Add/1 -> Saturation/1
  Saturation/1 -> Torque/1

== system a1_walking_backward/Stand Controller/Subsystem4 ==
  angle : Inport
  velocity : Inport  Port=2
  Add : Sum
  Constant1 : Constant  Value=-4
  Constant2 : Constant  Value=-40
  Constant3 : Constant  Value=-1
  Product : Product
  Product1 : Product
  Saturation : Saturate  UpperLimit=33.5  LowerLimit=-33.5
  Subtract : Sum  Inputs=+-
  Torque : Outport
  wires:
  angle/1 -> Subtract/1
  Constant2/1 -> Product/2
  Subtract/1 -> Product/1
  Constant1/1 -> Product1/2
  velocity/1 -> Product1/1
  Product1/1 -> Add/2
  Product/1 -> Add/1
  Constant3/1 -> Subtract/2
  Add/1 -> Saturation/1
  Saturation/1 -> Torque/1

== system a1_walking_backward/Stand Controller/Subsystem5 ==
  angle : Inport
  velocity : Inport  Port=2
  Add : Sum
  Constant1 : Constant  Value=-0.5
  Constant2 : Constant  Value=-5
  Constant3 : Constant  Value=0
  Product : Product
  Product1 : Product
  Saturation : Saturate  UpperLimit=33.5  LowerLimit=-33.5
  Subtract : Sum  Inputs=+-
  Torque : Outport
  wires:
  angle/1 -> Subtract/1
  Constant2/1 -> Product/2
  Subtract/1 -> Product/1
  Constant1/1 -> Product1/2
  velocity/1 -> Product1/1
  Product1/1 -> Add/2
  Product/1 -> Add/1
  Constant3/1 -> Subtract/2
  Add/1 -> Saturation/1
  Saturation/1 -> Torque/1

== system a1_walking_backward/Stand Controller/Subsystem6 ==
  angle : Inport
  velocity : Inport  Port=2
  Add : Sum
  Constant1 : Constant  Value=-2
  Constant2 : Constant  Value=-20
  Constant3 : Constant  Value=0
  Product : Product
  Product1 : Product
  Saturation : Saturate  UpperLimit=33.5  LowerLimit=-33.5
  Subtract : Sum  Inputs=+-
  Torque : Outport
  wires:
  angle/1 -> Subtract/1
  Constant2/1 -> Product/2
  Subtract/1 -> Product/1
  Constant1/1 -> Product1/2
  velocity/1 -> Product1/1
  Product1/1 -> Add/2
  Product/1 -> Add/1
  Constant3/1 -> Subtract/2
  Add/1 -> Saturation/1
  Saturation/1 -> Torque/1

== system a1_walking_backward/Stand Controller/Subsystem7 ==
  angle : Inport
  velocity : Inport  Port=2
  Add : Sum
  Constant1 : Constant  Value=-2
  Constant2 : Constant  Value=-20
  Constant3 : Constant  Value=0.5
  Product : Product
  Product1 : Product
  Saturation : Saturate  UpperLimit=33.5  LowerLimit=-33.5
  Subtract : Sum  Inputs=+-
  Torque : Outport
  wires:
  angle/1 -> Subtract/1
  Constant2/1 -> Product/2
  Subtract/1 -> Product/1
  Constant1/1 -> Product1/2
  velocity/1 -> Product1/1
  Product1/1 -> Add/2
  Product/1 -> Add/1
  Constant3/1 -> Subtract/2
  Add/1 -> Saturation/1
  Saturation/1 -> Torque/1

== system a1_walking_backward/Stand Controller/Subsystem8 ==
  angle : Inport
  velocity : Inport  Port=2
  Add : Sum
  Constant1 : Constant  Value=-2
  Constant2 : Constant  Value=-20
  Constant3 : Constant  Value=-1
  Product : Product
  Product1 : Product
  Saturation : Saturate  UpperLimit=33.5  LowerLimit=-33.5
  Subtract : Sum  Inputs=+-
  Torque : Outport
  wires:
  angle/1 -> Subtract/1
  Constant2/1 -> Product/2
  Subtract/1 -> Product/1
  Constant1/1 -> Product1/2
  velocity/1 -> Product1/1
  Product1/1 -> Add/2
  Product/1 -> Add/1
  Constant3/1 -> Subtract/2
  Add/1 -> Saturation/1
  Saturation/1 -> Torque/1

== system a1_walking_backward/Stand Controller/Subsystem9 ==
  angle : Inport
  velocity : Inport  Port=2
  Add : Sum
  Constant1 : Constant  Value=-0.5
  Constant2 : Constant  Value=-5
  Constant3 : Constant  Value=0
  Product : Product
  Product1 : Product
  Saturation : Saturate  UpperLimit=33.5  LowerLimit=-33.5
  Subtract : Sum  Inputs=+-
  Torque : Outport
  wires:
  angle/1 -> Subtract/1
  Constant2/1 -> Product/2
  Subtract/1 -> Product/1
  Constant1/1 -> Product1/2
  velocity/1 -> Product1/1
  Product1/1 -> Add/2
  Product/1 -> Add/1
  Constant3/1 -> Subtract/2
  Add/1 -> Saturation/1
  Saturation/1 -> Torque/1

== system a1_walking_backward/Walk Controller/Convert Forces to Torque1 ==
  F : Inport
  RR_Ang_Vec : Inport  Port=2
  RL_Ang_Vec : Inport  Port=3
  FL_Ang_Vec : Inport  Port=4
  FR_Ang_Vec : Inport  Port=5
  Force to Torque : MATLAB Function  TreatAsAtomicUnit=on
  Tau_FL : Outport
  Tau_RL : Outport  Port=2
  Tau_FR : Outport  Port=3
  Tau_RR : Outport  Port=4
  wires:
  F/1 -> Force to Torque/1(F)
  Force to Torque/1(Tau_RR) -> Tau_RR/1
  Force to Torque/2(Tau_FR) -> Tau_FR/1
  Force to Torque/3(Tau_FL) -> Tau_FL/1
  Force to Torque/4(Tau_RL) -> Tau_RL/1
  RR_Ang_Vec/1 -> Force to Torque/2(RR_ang_vec)
  RL_Ang_Vec/1 -> Force to Torque/3(RL_ang_vec)
  FL_Ang_Vec/1 -> Force to Torque/4(FL_ang_vec)
  FR_Ang_Vec/1 -> Force to Torque/5(FR_ang_vec)

== system a1_walking_backward/Walk Controller/Rigid Body Controller ==
  FL Pos : Inport
  RL Pos : Inport  Port=2
  FR Pos : Inport  Port=3
  RR Pos : Inport  Port=4
  COM_pos : Inport  Port=5
  COM_vel : Inport  Port=6
  COM_ang_vel : Inport  Port=7
  Rot : Inport  Port=8
  Clock : Clock
  Interpreted MATLAB Function : MATLABFcn  MATLABFcn=walking_forward_mpc(u)  OutputDimensions=12  Output1D=off
  Memory : Memory
  Mux : Mux  Inputs=9
  Rotation Matrix to Eul : MATLAB Function  TreatAsAtomicUnit=on
  Scope : Scope  NumInputPorts=5
  Selector : Selector  InputPortWidth=12  IndexOptions=Index vector (dialog)  Indices=[1 3]  OutputSizes=1
  Zero-Order Hold : ZeroOrderHold  SampleTime=.05
  u : Outport
  wires:
  COM_pos/1 -> Mux/1
  COM_vel/1 -> Mux/2
  COM_ang_vel/1 -> Mux/4
  FL Pos/1 -> Mux/5
  RL Pos/1 -> Mux/6
  FR Pos/1 -> Mux/7
  RR Pos/1 -> Mux/8
  Rot/1 -> Rotation Matrix to Eul/1(u)
  Rotation Matrix to Eul/1(y) -> Mux/3
  Interpreted MATLAB Function/1 -> Memory/1
  Memory/1 -> Selector/1, u/1
  Mux/1 -> Zero-Order Hold/1
  Zero-Order Hold/1 -> Interpreted MATLAB Function/1
  Clock/1 -> Mux/9
  Selector/1 -> Scope/1

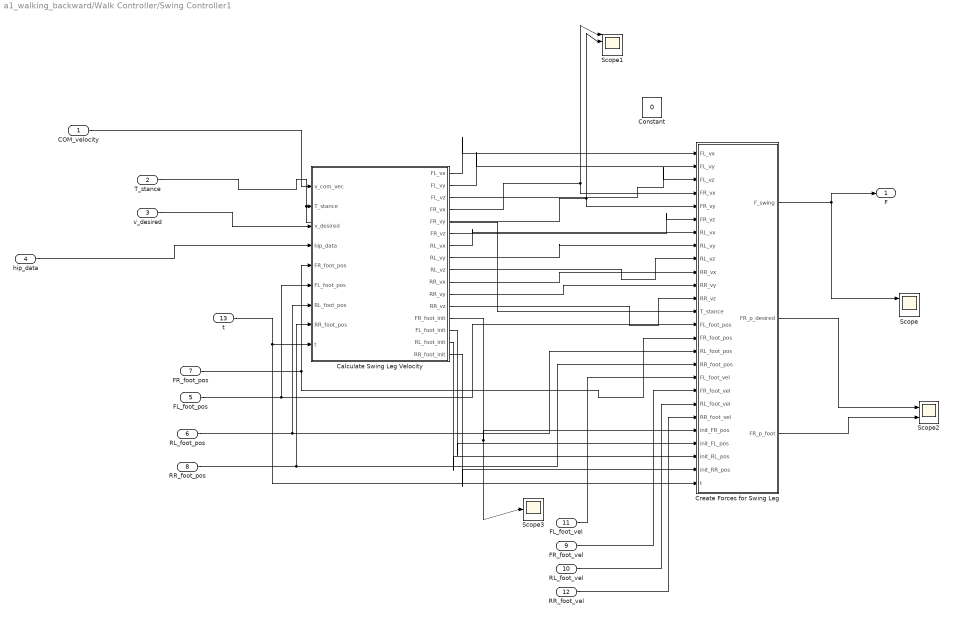
== system a1_walking_backward/Walk Controller/Swing Controller1 ==
  COM_velocity : Inport
  T_stance : Inport  Port=2
  v_desired : Inport  Port=3
  hip_data : Inport  Port=4
  FL_foot_pos : Inport  Port=5
  RL_foot_pos : Inport  Port=6
  FR_foot_pos : Inport  Port=7
  RR_foot_pos : Inport  Port=8
  FR_foot_vel : Inport  Port=9
  RL_foot_vel : Inport  Port=10
  FL_foot_vel : Inport  Port=11
  RR_foot_vel : Inport  Port=12
  t : Inport  Port=13
  Calculate Swing Leg Velocity : MATLAB Function  TreatAsAtomicUnit=on  SystemSampleTime=0.2
  Constant : Constant  Value=0
  Create Forces for Swing Leg : MATLAB Function  TreatAsAtomicUnit=on
  Scope : Scope  NumInputPorts=3
  Scope1 : Scope  NumInputPorts=4
  Scope2 : Scope  NumInputPorts=2
  Scope3 : Scope
  F : Outport
  wires:
  T_stance/1 -> Create Forces for Swing Leg/13(T_stance), Calculate Swing Leg Velocity/2(T_stance)
  v_desired/1 -> Calculate Swing Leg Velocity/3(v_desired)
  Create Forces for Swing Leg/1(F_swing) -> Scope/1, F/1
  t/1 -> Calculate Swing Leg Velocity/9(t), Create Forces for Swing Leg/26(t)
  hip_data/1 -> Calculate Swing Leg Velocity/4(hip_data)
  Calculate Swing Leg Velocity/12(RR_vz) -> Create Forces for Swing Leg/12(RR_vz)
  Calculate Swing Leg Velocity/11(RR_vy) -> Create Forces for Swing Leg/11(RR_vy)
  Calculate Swing Leg Velocity/10(RR_vx) -> Create Forces for Swing Leg/10(RR_vx)
  Calculate Swing Leg Velocity/9(RL_vz) -> Create Forces for Swing Leg/9(RL_vz)
  Calculate Swing Leg Velocity/8(RL_vy) -> Create Forces for Swing Leg/8(RL_vy)
  Calculate Swing Leg Velocity/7(RL_vx) -> Create Forces for Swing Leg/7(RL_vx)
  Calculate Swing Leg Velocity/6(FR_vz) -> Create Forces for Swing Leg/6(FR_vz)
  Calculate Swing Leg Velocity/5(FR_vy) -> Create Forces for Swing Leg/5(FR_vy), Scope1/2
  Calculate Swing Leg Velocity/4(FR_vx) -> Create Forces for Swing Leg/4(FR_vx), Scope1/1
  Calculate Swing Leg Velocity/3(FL_vz) -> Create Forces for Swing Leg/3(FL_vz)
  Calculate Swing Leg Velocity/2(FL_vy) -> Create Forces for Swing Leg/2(FL_vy)
  Calculate Swing Leg Velocity/1(FL_vx) -> Create Forces for Swing Leg/1(FL_vx)
  FR_foot_pos/1 -> Create Forces for Swing Leg/15(FR_foot_pos), Calculate Swing Leg Velocity/5(FR_foot_pos)
  RL_foot_pos/1 -> Calculate Swing Leg Velocity/7(RL_foot_pos), Create Forces for Swing Leg/16(RL_foot_pos)
  RR_foot_pos/1 -> Create Forces for Swing Leg/17(RR_foot_pos), Calculate Swing Leg Velocity/8(RR_foot_pos)
  FL_foot_vel/1 -> Create Forces for Swing Leg/18(FL_foot_vel)
  FR_foot_vel/1 -> Create Forces for Swing Leg/19(FR_foot_vel)
  RL_foot_vel/1 -> Create Forces for Swing Leg/20(RL_foot_vel)
  RR_foot_vel/1 -> Create Forces for Swing Leg/21(RR_foot_vel)
  Create Forces for Swing Leg/2(FR_p_desired) -> Scope2/1
  COM_velocity/1 -> Calculate Swing Leg Velocity/1(v_com_vec)
  Calculate Swing Leg Velocity/13(FR_foot_init) -> Scope3/1, Create Forces for Swing Leg/22(init_FR_pos)
  Create Forces for Swing Leg/3(FR_p_foot) -> Scope2/2
  FL_foot_pos/1 -> Calculate Swing Leg Velocity/6(FL_foot_pos), Create Forces for Swing Leg/14(FL_foot_pos)
  Calculate Swing Leg Velocity/14(FL_foot_init) -> Create Forces for Swing Leg/23(init_FL_pos)
  Calculate Swing Leg Velocity/15(RL_foot_init) -> Create Forces for Swing Leg/24(init_RL_pos)
  Calculate Swing Leg Velocity/16(RR_foot_init) -> Create Forces for Swing Leg/25(init_RR_pos)

== matlab function a1_walking_backward/Rear Right Leg/Separate Torques ==
  data: torque_vector input; hip_torque output; thigh_torque output; calf_torque output
function [hip_torque, thigh_torque, calf_torque] = fcn(torque_vector)

hip_torque = torque_vector(1);
thigh_torque = torque_vector(2);
calf_torque = torque_vector(3);

== matlab function a1_walking_backward/Front Left Leg/Separate Torques ==
  data: torque_vector input; hip_torque output; thigh_torque output; calf_torque output
function [hip_torque, thigh_torque, calf_torque] = fcn(torque_vector)

hip_torque = torque_vector(1);
thigh_torque = torque_vector(2);
calf_torque = torque_vector(3);

== matlab function a1_walking_backward/Stand Controller/MATLAB Function ==
  data: angle_vector input; hip_angle output; thigh_angle output; calf_angle output
function [hip_angle, thigh_angle, calf_angle] = fcn(angle_vector)

hip_angle = angle_vector(1);
thigh_angle = angle_vector(2);
calf_angle = angle_vector(3);

== matlab function a1_walking_backward/Stand Controller/MATLAB Function1 ==
  data: velocity_vector input; hip_velocity output; thigh_velocity output; calf_velocity output
function [hip_velocity, thigh_velocity, calf_velocity] = fcn(velocity_vector)

hip_velocity = velocity_vector(1);
thigh_velocity = velocity_vector(2);
calf_velocity = velocity_vector(3);

== matlab function a1_walking_backward/Stand Controller/MATLAB Function2 ==
  data: angle_vector input; hip_angle output; thigh_angle output; calf_angle output
function [hip_angle, thigh_angle, calf_angle] = fcn(angle_vector)

hip_angle = angle_vector(1);
thigh_angle = angle_vector(2);
calf_angle = angle_vector(3);

== matlab function a1_walking_backward/Stand Controller/MATLAB Function3 ==
  data: velocity_vector input; hip_velocity output; thigh_velocity output; calf_velocity output
function [hip_velocity, thigh_velocity, calf_velocity] = fcn(velocity_vector)

hip_velocity = velocity_vector(1);
thigh_velocity = velocity_vector(2);
calf_velocity = velocity_vector(3);

== matlab function a1_walking_backward/Stand Controller/MATLAB Function4 ==
  data: angle_vector input; hip_angle output; thigh_angle output; calf_angle output
function [hip_angle, thigh_angle, calf_angle] = fcn(angle_vector)

hip_angle = angle_vector(1);
thigh_angle = angle_vector(2);
calf_angle = angle_vector(3);

== matlab function a1_walking_backward/Stand Controller/MATLAB Function5 ==
  data: velocity_vector input; hip_velocity output; thigh_velocity output; calf_velocity output
function [hip_velocity, thigh_velocity, calf_velocity] = fcn(velocity_vector)

hip_velocity = velocity_vector(1);
thigh_velocity = velocity_vector(2);
calf_velocity = velocity_vector(3);

== matlab function a1_walking_backward/Stand Controller/MATLAB Function6 ==
  data: angle_vector input; hip_angle output; thigh_angle output; calf_angle output
function [hip_angle, thigh_angle, calf_angle] = fcn(angle_vector)

hip_angle = angle_vector(1);
thigh_angle = angle_vector(2);
calf_angle = angle_vector(3);

== matlab function a1_walking_backward/Stand Controller/MATLAB Function7 ==
  data: velocity_vector input; hip_velocity output; thigh_velocity output; calf_velocity output
function [hip_velocity, thigh_velocity, calf_velocity] = fcn(velocity_vector)

hip_velocity = velocity_vector(1);
thigh_velocity = velocity_vector(2);
calf_velocity = velocity_vector(3);

== matlab function a1_walking_backward/Walk Controller/Combine Forces ==
  data: t input; F output; rigid_body_forces input; swing_forces input
function F = fcn(t, rigid_body_forces, swing_forces)
%#codegen
intervals = 0:0.2:5;

interval_idx = discretize(t, intervals);

if mod(interval_idx(1), 2) == 0
    F = [rigid_body_forces(1:3); -swing_forces(4:6); -swing_forces(7:9); rigid_body_forces(10:12)];
else
    F = [-swing_forces(1:3); rigid_body_forces(4:6); rigid_body_forces(7:9); -swing_forces(10:12)];
end

== matlab function a1_walking_backward/Walk Controller/Rigid Body Controller/Rotation Matrix to Eul ==
  data: u input; y output
function y = fcn(u)
y = rotm2eul(u);
